simulink model "p560Progetto_jacobiano"  (R2020b)
settings: Solver=VariableStepAuto  StartTime=0.0  StopTime=30  RelTol=1e-3
undefined symbols (not defined in the file or in its folder): DiscIntNeverNeededParam, qn
libraries: roblocks x6
settings Model: PacingRate=32  OrderedModelArguments=off  Creator=Valentina  LastModifiedBy=Valentina

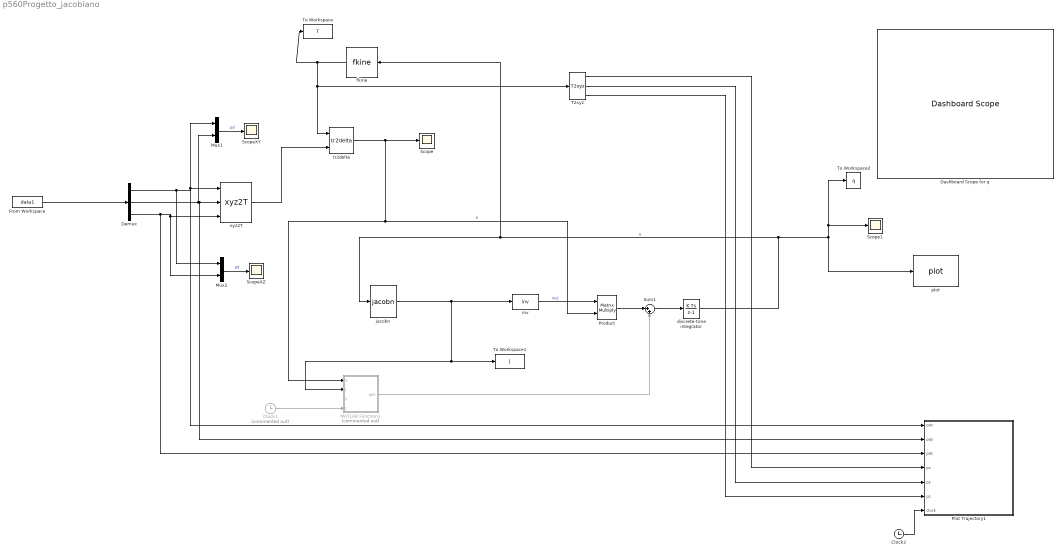
== system p560Progetto_jacobiano ==
  Clock1 : Clock  Commented=on
  Clock2 : Clock
  Dashboard Scope for q : DashboardScope
  Demux : Demux  Outputs=3
  From Workspace : FromWorkspace  VariableName=data1  SampleTime=-1
  MATLAB Function1 : MATLAB Function  Priority=6  Commented=on  TreatAsAtomicUnit=on
  Mux1 : Mux  Inputs=2
  Mux2 : Mux  Inputs=2
  Plot Trajectory1 : MATLAB Function  TreatAsAtomicUnit=on  SystemSampleTime=0.3
  Product : Product  Multiplication=Matrix(*)  InputSameDT=on  RndMeth=Zero  SaturateOnIntegerOverflow=on  OutDataTypeStr=Inherit: Same as first input
  Scope : Scope
  Scope1 : Scope
  ScopeXY : Scope
  ScopeXZ : Scope
  Sum1 : Sum  Inputs=|++
  T2xyz : roblocks/Toolbox/T2xyz
  To Workspace : ToWorkspace  VariableName=T  SampleTime=-1
  To Workspace1 : ToWorkspace  VariableName=J  SampleTime=-1
  To Workspace2 : ToWorkspace  VariableName=q  SampleTime=-1
  discrete-time integrator : DiscreteIntegrator  gainval=5  InitialCondition=qn  SampleTime=0.05  ICPrevOutput=DiscIntNeverNeededParam  ICPrevScaledInput=DiscIntNeverNeededParam
  fkine : roblocks/Arm/fkine  robot=p560
  inv : MATLABFcn  MATLABFcn=inv  Output1D=off
  jacobn : roblocks/Arm/jacobn  robot=p560
  plot : roblocks/Arm/plot  robot=p560  fps=5  holdplot=on
  tr2delta : roblocks/Toolbox/tr2delta
  xyz2T : roblocks/Toolbox/xyz2T
  wires:
  jacobn/1 -> To Workspace1/1, MATLAB Function1/2(J), inv/1
  inv/1 -> Product/1  "invJ"
  discrete-time integrator/1 -> fkine/1, jacobn/1, plot/1, Scope1/1, To Workspace2/1  "q"
  xyz2T/1 -> tr2delta/2
  fkine/1 -> To Workspace/1, tr2delta/1, T2xyz/1
  Demux/2 -> Mux1/2, Plot Trajectory1/2(pdy), xyz2T/2
  Demux/1 -> Mux1/1, Plot Trajectory1/1(pdx), xyz2T/1, Mux2/1
  Demux/3 -> Plot Trajectory1/3(pdz), Mux2/2, xyz2T/3
  tr2delta/1 -> Scope/1, Product/2, MATLAB Function1/1(e)  "e"
  Clock1/1 -> MATLAB Function1/4(t)
  MATLAB Function1/1(qp2) -> Sum1/2
  Product/1 -> Sum1/1
  Sum1/1 -> discrete-time integrator/1
  Clock2/1 -> Plot Trajectory1/7(clock)
  T2xyz/1 -> Plot Trajectory1/4(px)
  T2xyz/2 -> Plot Trajectory1/5(py)
  Mux2/1 -> ScopeXZ/1  "pd"
  Mux1/1 -> ScopeXY/1  "pd"
  T2xyz/3 -> Plot Trajectory1/6(pz)
  From Workspace/1 -> Demux/1

== matlab function p560Progetto_jacobiano/Plot Trajectory1 ==
  settings: updateMethod=DISCRETE
  data: pdx input; pdy input; pdz input; px input; py input; pz input; clock input
function PlotTraiettoria(pdx,pdy,pdz,px,py,pz, clock)

eml.extrinsic('findobj','get','set','figure','clf',...
              'hold','delete','plot','axis','grid',...
              'hggroup','quiver','drawnow');
          
persistent target;
% persistent chain;
% persistent velocity;
% persistent chain2;
persistent i;
persistent k;

persistent obiettivo;


n=1;


if isempty(target)
    target=zeros(n,1);
    i=0;
    
end

if isempty(obiettivo)
    obiettivo=zeros(n,1);
    k=0;
end


i=i+1;
if i>n
    i=1;
end

k=k+1;
if k>n
    k=1;
end

%           
% pex=[0;...
%     cos(theta1);...
%     cos(theta1)+cos(theta1+theta2);...
%     cos(theta1)+cos(theta1+theta2)+cos(theta1+theta2+theta3)];
% 
% pey=[0;...
%     sin(theta1);...
%     sin(theta1)+sin(theta1+theta2);...
%     sin(theta1)+sin(theta1+theta2)+sin(theta1+theta2+theta3)];
% 
% 
% pex2=[0;...
%     cos(th1);...
%     cos(th1)+cos(th1+th2);...
%     cos(th1)+cos(th1+th2)+cos(th1+th2+th3)];
% 
% pey2=[0;...
%     sin(th1);...
%     sin(th1)+sin(th1+th2);...
%     sin(th1)+sin(th1+th2)+sin(th1+th2+th3)];
% 
% 
%           
foundFig=findobj('Tag','trajScope');
    
if ~isempty(foundFig) & (clock==1)
    delete(foundFig)
    foundFig=findobj('Tag','trajScope');  
end


 if isempty(foundFig)
    fig=figure('Color','white');
    clf(fig);
    set(fig,'Name','Trajectory');
    set(fig,'DoubleBuffer','on','Tag','trajScope');
    set(fig,'Renderer','painters');
    hold('on');
    hax=get(fig,'CurrentAxes');
    set(hax,'DrawMode','fast','Box','off');    
    
    target(i)=plot3(hax,pdx,pdy,pdz,'bo','MarkerFaceColor','#4DBEEE');
  
 else
    hax=get(foundFig,'CurrentAxes');

end
% 
j=i-(n-1);
if j<=0
    j=j+n;
end

if target(j)~=0
    delete(target(j));
end

% draw the desired point
target(i)=plot3(pdx,pdy,pdz,'bo','MarkerFaceColor','#4DBEEE');
target(k)=plot3(px,py,pz,'rh','MarkerFaceColor','r');


grid('on');
axis([-1 1 -1 1 -1 1])
drawnow;

== matlab function p560Progetto_jacobiano/MATLAB Function1 ==
  settings: updateMethod=DISCRETE
  data: e input; J input; qp2 output size=6; k input; t input
function qp2 = fcn(e,J,k, t)

persistent f_v
persistent e_v
persistent last_k

n=400;

if isempty(last_k)
    last_k=-1;
end


if isempty(f_v)
    f_v=zeros(n,3);
end
   
if isempty(e_v)
    e_v=zeros(n,2);
end


if k~=last_k
%   
     %disp(k)
     last_k=k;
     
     if t<500
        f_v(k,:)=0.6.*f_v(k,:)+(pinv(J).*e_v(k,:)')';
     else
        f_v(k,:)=0.95.*f_v(k,:)+(pinv(J).*e_v(k,:)')';
     end
     
     
     e_v(k,:)=e';
%     
%  
end


qp2=f_v(k,:)';
